simulink model "UDP_transceiver"  (R2022b)
settings: Solver=VariableStepAuto  StartTime=0.0  StopTime=10.0  RelTol=1e-3
libraries: slrealtimeiplib x2, slrealtimeutilitieslib x1, etargetslib x1
settings Model: Creator=lcx19  LastModifiedBy=lcx19

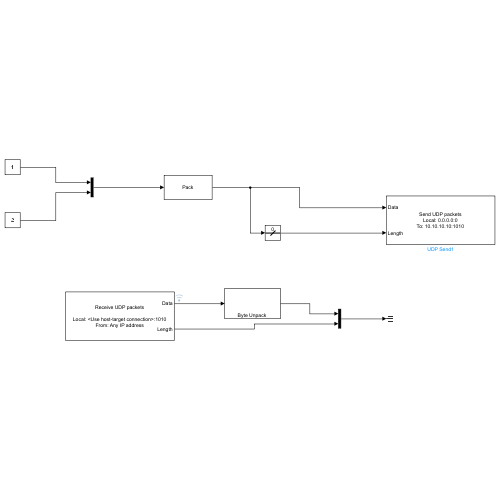
[thumbnail: Simulink's stored preview of the top-level diagram]
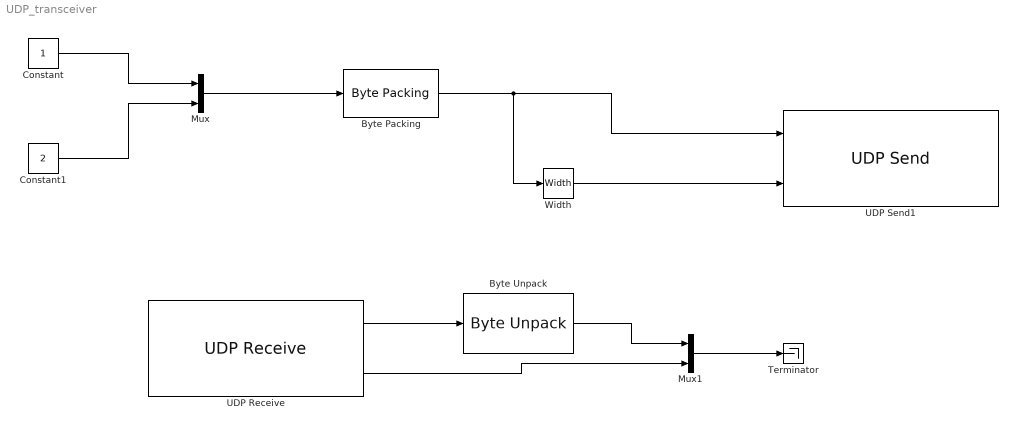
== system UDP_transceiver ==
  Byte Packing : slrealtimeutilitieslib/Byte Packing  MaskPackedDataType=uint8  MaskUnpackedDataTypes={'uint8'}  MaskAlignment=1
  Byte Unpack : etargetslib/Byte Unpack  dimensions={[2]}  datatypes={'double'}  byteAlign=1
      settings: LibrarySourceBlock=embeddedtargetslib/Host Communication/Byte Unpack
  Constant : Constant  OutDataTypeStr=uint8
  Constant1 : Constant  Value=2  OutDataTypeStr=uint8
  Mux : Mux  Inputs=2
  Mux1 : Mux  Inputs=2
  Terminator : Terminator
  UDP Receive : slrealtimeiplib/UDP Receive  useHostTargetConn=on  ipAddress=10.10.10.10  localPort=1010  rcvWidth=16  rcvFmAny=on  fmAddress='10.10.10.10'  sampleTime=-1  enableMessage=off  maxPackets=1
  UDP Send1 : slrealtimeiplib/UDP Send  useHostTargetConn=off  toAddress='10.10.10.10'  toPort=1010  sampleTime=Ts  enableMessage=off
  Width : Width
  wires:
  Constant/1 -> Mux/1
  Constant1/1 -> Mux/2
  Mux/1 -> Byte Packing/1
  Byte Packing/1 -> Width/1, UDP Send1/1
  Width/1 -> UDP Send1/2
  UDP Receive/1 -> Byte Unpack/1
  Byte Unpack/1 -> Mux1/1
  UDP Receive/2 -> Mux1/2
  Mux1/1 -> Terminator/1
